simulink library "tqd"  (R2021b)
settings: Solver=VariableStepAuto  StartTime=0.0  StopTime=10.0  RelTol=1e-3
undefined symbols (not defined in the file or in its folder): ATQD_APSDecReq_X_kph, ATQD_APSDecReq_Y_mps2, ATQD_APSDecReqCMD_X_kph, ATQD_APSDecReqTs_X_pct, ATQD_APSDecTimeGain_X_Deg, ATQD_APSDecTimeGain_Y_s, ATQD_APSReqLowSpd_X_Deg, ATQD_AutoHoldReleaseBPS_X_Deg, ATQD_AWDLoadTrqnsGain_X_kg, ATQD_AWDLoadTrqnsGain_Y_pct, ATQD_BOSEnBPSPosn_X_kph, ATQD_BOSMap_X_rpm, ATQD_BOSMap_Y_pct, ATQD_CreepBaseTqD_X_kph, ATQD_CreepBaseTqD_Y_Deg, ATQD_CreepBaseTqR_X_kph, ATQD_CreepBaseTqR_Y_Deg, ATQD_CreepBPSDisPosn_X_Deg, ATQD_CreepBPSDisPosnR_X_Deg, ATQD_CreepBPSEnPosn_X_Deg, ATQD_CreepBPSEnPosnR_X_Deg, ATQD_CreepDeltaTq_X_kph, ATQD_CreepIterm_X_kph, ATQD_CreepIterm_Y_kph, ATQD_CreepItermMaxLimit_X_pct, ATQD_CreepPreloadTime_X_kph, ATQD_CreepPreloadTq_X_kph, ATQD_CreepPreloadTq_Y_s, ATQD_CreepProtTq_X_Deg, ATQD_CreepPterm_X_kph, ATQD_CreepPterm_Y_kph, ATQD_ECOTqMapD_X_rpm, ATQD_ECOTqMapD_Y_pct, ATQD_EOPDTqMapDCon_X_rpm, ATQD_EOPDTqMapDCon_Y_Deg, ATQD_EstInitVehWeight_X_c, ATQD_LHMRollGenMapD_X_rpm, ATQD_LHMRollGenMapD_Y_rpm, ATQD_LHMTqMapD_X_rpm, ATQD_LHMTqMapD_Y_pct, ATQD_NL1TqMapD_X_rpm, ATQD_NL1TqMapD_Y_pct, ATQD_NOPDTqMapDCon_X_rpm, ATQD_NOPDTqMapDCon_Y_Deg, ATQD_NRMRrEDUSpRat_X_rpm, ATQD_NRMRrEDUSpRat_Y_Nm, ATQD_OPDHoldDownRelDelay_X_Deg, ATQD_OPDHoldEnSpd_X_Deg, ATQD_OPDHoldRelDetTime_X_Deg, ATQD_OPDHoldReleaseTq_X_Deg, ATQD_OrigPedTqLowLim_X_Deg, ATQD_OrigPedTqLowLim_Y_pct, ATQD_PedalMapClimbUpLim_X_rpm, ATQD_PedalMapClimbUpLim_Y_Deg, ATQD_PreLoadTq_X_s, ATQD_RollGenMapEL1_X_rpm, ATQD_RollGenMapEL1_Y_rpm, ATQD_SL1TqMapD_X_rpm, ATQD_SL1TqMapD_Y_pct, ATQD_SlideRegenTqGain_X_Gps ... (+487)
libraries: hcu_lib x83, simulink x73, tqr x1
(part 13 of 19)

== system tqd/TQD/TorqueDemand/Signal_convert/SWC2_Subsystem/Speed Setting Mode/MSA Speed Setting ON ==
  note: MSA SPEED SETTING MODE
  VVMC_MSACrlSta_enum : Inport
  "VTQD_SWC2ScrollUpSta_enum  " : Inport  Port=2
  "VTQD_SWC2ScrollDownSta_enum  " : Inport  Port=3
  VTQD_SpdLim4SetSpd_raw32 : Inport  Port=4
  VTQD_SetSpdDeltaLongFit_kph : Inport  Port=5
  VINP_Distanceunit_flg : Inport  Port=6
  VTQD_SWC2ResUpSta_flg : Inport  Port=7
  VTQD_SWC2SetDownSta_flg : Inport  Port=8
  VINP_SmartEcoModeSW_flg : Inport  Port=9
  VINP_IVIACCAdaptiveSta_flg : Inport  Port=10
  VTQD_Set2MeterSpd_flg : Inport  Port=11
  VTQD_SetRoadSpdLim_flg : Inport  Port=12
  VINP_ADASSLIFSpdLim_enum : Inport  Port=13
  VTQD_LScrollPressShort_flg : Inport  Port=14
  VVMC_MeterIndSpeed_raw32 : Inport  Port=15
  Action Port : ActionPort  InitializeStates=reset
  " 1" : Constant  Value=KTQD_MSAActiveMetSpdLoMPH_mph
  " 80" : Constant  Value=KTQD_MSAActiveMetSpdLo_kph
  1 : Constant  Value=KTQD_SetSpdDeltaShort_kph
  160 : Constant  Value=KTQD_MSAActiveMetSpdHi_kph
  2 : Constant  Value=KTQD_MSAActiveMetSpdHiMPH_mph
  3 : Constant  Value=KTQD_SetSpdDeltaLongMPH_mph
  4 : Constant  Value=KTQD_SmartEcoLimitSpd_mph
  5 : Constant  Value=KTQD_SetSpdDeltaLong_kph
  6 : Constant  Value=KTQD_SmartEcoLimitSpd_kph
  AND : Logic  AllPortsSameDT=off  OutDataTypeStr=boolean
  AND1 : Logic  AllPortsSameDT=off  OutDataTypeStr=boolean
  Cast To Single : DataTypeConversion  OutDataTypeStr=int8
  Delta Long Fit Base : Constant  Value=KTQD_SetSpdDeltaLongFit_kph
  KTQD_ISATestSW_flg : Constant  Value=KTQD_ISATestSW_flg
  MSA : Stateflow chart  TreatAsAtomicUnit=on
      settings: PortSchema="{\"entries\":[{\"content\":{\"sides\":[{\"content\":{\"connectorIds\":[\"In9\",\"In6\",\"In3\",\"In5\",\"In7\",\"In8\",\"In1\",\"In2\",\"In12\",\"In13\",\"In14\",\"In10\",\"In11\",\"In4\"]},\"type\":\"ConnectorPlacement.EquallySpacedRectSide\",\"uuid\":\"4fee65fe-2e32-4dfc-9c8c-ef7087e97952\"},{\"content\":{\"connectorIds\":[\"Out1\"],\"side\":\"RIGHT\"},\"type\":\"ConnectorPlacement.EquallySpacedRectSide\",\"uuid\":\"8d915692-cb0b-4a06-a57e-690cea51e532\"},{\"content\":{\"connectorIds\":[],\"side\":\"TOP\"},\"type\":\"ConnectorPlacement.EquallySpacedRectSide\",\"uuid\":\"3fa43362-4ddf-4693-9d82-d4f790f00c9c\"}]},\"type\":\"ConnectorPlacement.EquallySpacedConnector\",\"uuid\":\"c1a6cfdc-58f2-45b0-af62-575976a00cf2\"}],\"packageUris\":[\"http://schema.mathworks.com/mf0/Connector/R2020b\"],\"version\":\"1.0\"}"
  MSASetSpd_241018 : Stateflow chart  TreatAsAtomicUnit=on
  ONE : Constant  Value=ONE_INT
  Relational Operator2 : RelationalOperator  Operator===  OutDataTypeStr=boolean  RndMeth=Simplest
  Relational Operator4 : RelationalOperator  Operator===  OutDataTypeStr=boolean  RndMeth=Simplest
  Round : Rounding  Operator=round
  Specific_STATE_ChangeToOFF : Stateflow chart  TreatAsAtomicUnit=on
  Switch{,1..5,7} (7 alike) : Switch  Criteria=u2 > Threshold
  standby : Constant  Value=ENUM_ADASMSASTA_STANDBY
  standby1 : Constant  Value=KTQD_MSASetSpdSource_flg
  zero : Constant  Value=ZERO_INT
  VSCP_MSASetSpd_kph : Outport
  wires:
  VTQD_SpdLim4SetSpd_raw32/1 -> [VTQD_SpdLim4SetSpd_raw32]
  Delta Long Fit Base/1 -> MSA/11(KTQD_SetSpdDeltaLongFit_kph)
  Switch2/1 -> [VTQD_MSAActiveMetSpdHi_raw32]  "VTQD_MSAActiveMetSpdHi_raw32"
  Switch3/1 -> [VTQD_MSAActiveMetSpdLo_raw32]  "VTQD_MSAActiveMetSpdLo_raw32"
  VVMC_MSACrlSta_enum/1 -> [VVMC_MSACrlSta_enum]
  1/1 -> MSA/2(KTQD_SetSpdDeltaShort_kph)
  "VTQD_SWC2ScrollDownSta_enum  "/1 -> [VTQD_SWC2ScrollDownSta_enum]
  "VTQD_SWC2ScrollUpSta_enum  "/1 -> [VTQD_SWC2ScrollUpSta_enum]
  Specific_STATE_ChangeToOFF/1(VTQD_ChangeToOFF_flg) -> [VTQD_ChangeToOFF_flg]
  [VVMC_MSACrlSta_enum] -> Specific_STATE_ChangeToOFF/1(VINP_MSACrlSta_enum)
  AND1/1 -> Switch1/2
  zero/1 -> Relational Operator4/2
  standby/1 -> Relational Operator2/2
  ONE/1 -> Switch1/1
  Cast To Single/1 -> Relational Operator4/1, Switch1/3
  Relational Operator2/1 -> AND1/1
  [VVMC_MSACrlSta_enum] -> Relational Operator2/1
  Relational Operator4/1 -> AND1/2
  Switch1/1 -> VSCP_MSASetSpd_kph/1
  [VINP_Distanceunit_flg] -> Switch2/2
  VINP_Distanceunit_flg/1 -> [VINP_Distanceunit_flg]
  [VINP_Distanceunit_flg] -> Switch3/2
  " 80"/1 -> Switch3/3
  " 1"/1 -> Switch3/1
  [VINP_Distanceunit_flg] -> Switch4/2
  5/1 -> Switch4/3
  3/1 -> Switch4/1
  Round/1 -> Cast To Single/1
  VINP_SmartEcoModeSW_flg/1 -> [VINP_SmartEcoModeSW_flg]
  [VINP_SmartEcoModeSW_flg] -> Switch/2
  160/1 -> Switch/3
  Switch/1 -> Switch2/3
  [VINP_SmartEcoModeSW_flg] -> Switch5/2
  2/1 -> Switch5/3
  Switch5/1 -> Switch2/1
  4/1 -> Switch5/1
  6/1 -> Switch/1
  [VTQD_ChangeToOFF_flg] -> MSA/3(VTQD_ChangeToOFF_flg)
  [VVMC_MSACrlSta_enum] -> MSASetSpd_241018/1(VVMC_MSACrlSta_enum)
  AND/1 -> MSASetSpd_241018/2(VINP_IVIACCAdaptiveSta_flg)
  KTQD_ISATestSW_flg/1 -> AND/2
  [VTQD_SpdLim4SetSpd_raw32] -> MSASetSpd_241018/3(VTQD_SpdLim4SetSpd_raw32)
  [VTQD_MSAActiveMetSpdHi_raw32] -> MSASetSpd_241018/4(VTQD_MSAActiveMetSpdHi_raw32)
  [VTQD_MSAActiveMetSpdLo_raw32] -> MSASetSpd_241018/5(VTQD_MSAActiveMetSpdLo_raw32)
  [VTQD_SWC2ScrollUpSta_enum] -> MSASetSpd_241018/7(VTQD_SWC2ScrollUpSta_enum)
  [VTQD_SWC2ScrollDownSta_enum] -> MSASetSpd_241018/8(VTQD_SWC2ScrollDownSta_enum)
  [VINP_Distanceunit_flg] -> MSASetSpd_241018/11(VINP_Distanceunit_flg)
  MSASetSpd_241018/1(VTQD_MSASetSpd_raw32) -> [VTQD_MSASetSpd_raw32]  "VTQD_MSASetSpd_raw32"
  standby1/1 -> Switch7/2
  [VTQD_MSASetSpd_raw32] -> Switch7/1
  Switch7/1 -> Round/1
  VTQD_SetSpdDeltaLongFit_kph/1 -> [VTQD_SetSpdDeltaLongFit_kph]
  VTQD_SWC2ResUpSta_flg/1 -> [VTQD_SWC2ResUpSta_flg]
  Switch4/1 -> [VTQD_SetSpdDeltaLong_kph]  "VTQD_SetSpdDeltaLong_kph"
  VTQD_SWC2SetDownSta_flg/1 -> [VTQD_SWC2SetDownSta_flg]
  VINP_IVIACCAdaptiveSta_flg/1 -> [VINP_IVIACCAdaptiveSta_flg]
  [VINP_IVIACCAdaptiveSta_flg] -> AND/1
  VTQD_Set2MeterSpd_flg/1 -> [VTQD_Set2MeterSpd_flg]
  [VTQD_Set2MeterSpd_flg] -> MSASetSpd_241018/6(VTQD_Set2MeterSpd_flg)
  VTQD_SetRoadSpdLim_flg/1 -> [VTQD_SetRoadSpdLim_flg]
  [VTQD_SetRoadSpdLim_flg] -> MSASetSpd_241018/10(VTQD_SetRoadSpdLim_flg)
  VINP_ADASSLIFSpdLim_enum/1 -> [VINP_ADASSLIFSpdLim_enum]
  [VINP_ADASSLIFSpdLim_enum] -> MSASetSpd_241018/12(VTQD_ADASSLIFSpdLimDet_flg)
  VTQD_LScrollPressShort_flg/1 -> [VTQD_LScrollPressShort_flg]
  [VTQD_LScrollPressShort_flg] -> MSASetSpd_241018/13(VTQD_LScrollPressShort_flg)
  VVMC_MeterIndSpeed_raw32/1 -> [VVMC_MeterIndSpeed_raw32]
  [VVMC_MeterIndSpeed_raw32] -> MSASetSpd_241018/14(VVMC_MeterIndSpeed_raw32)
  [VTQD_SetSpdDeltaLong_kph] -> MSASetSpd_241018/9(VTQD_SetSpdDeltaLong_raw32)
  [VVMC_MSACrlSta_enum] -> MSA/9(VVMC_MSACrlSta_enum)
  [VTQD_SpdLim4SetSpd_raw32] -> MSA/6(VVMC_MeterIndSpeed_raw32)
  [VINP_Distanceunit_flg] -> MSA/5(VINP_Distanceunit_flg)
  [VTQD_MSAActiveMetSpdHi_raw32] -> MSA/7(KTQD_MSAActiveMetSpdHi_raw32)
  [VTQD_MSAActiveMetSpdLo_raw32] -> MSA/8(KTQD_MSAActiveMetSpdLo_raw32)
  [VTQD_SetSpdDeltaLong_kph] -> MSA/1(KTQD_SetSpdDeltaLong_kph)
  [VTQD_SWC2ScrollUpSta_enum] -> MSA/12(VTQD_SWC2ScrollUpSta_enum)
  [VTQD_SWC2ResUpSta_flg] -> MSA/13(VTQD_SWC2ResUpSta_flg)
  [VTQD_SWC2SetDownSta_flg] -> MSA/14(VTQD_SWC2SetDownSta_flg)
  [VTQD_SetSpdDeltaLongFit_kph] -> MSA/10(VTQD_SetSpdDeltaLongFit_kph)
  [VTQD_SWC2ScrollDownSta_enum] -> MSA/4(VTQD_SWC2ScrollDownSta_enum)
  MSA/1(VTQD_MSASetSpd_kph) -> [VTQD_MSASetSpd_kph]  "VTQD_MSASetSpd_kph"
  [VTQD_MSASetSpd_kph] -> Switch7/3

== system tqd/TQD/TorqueDemand/Signal_convert/SWC2_Subsystem/Speed Setting Mode/SWC2ScrollDownSta ==
  note: Long press or Short press
  INPUT : Inport
  task_time_s : Inport  Port=2
  AND : Logic  AllPortsSameDT=off  OutDataTypeStr=boolean
  AND1 : Logic  AllPortsSameDT=off  OutDataTypeStr=boolean
  Constant1 : Constant  Value=ENUM_SWCBOTTONPRESS_LONGPRESS
  Constant2 : Constant  Value=KTQD_ScrollDownShortPLim_s
  Constant3 : Constant  Value=KTQD_ScrollDownLongPLim_s
  Constant7 : Constant  Value=ENUM_SWCBOTTONPRESS_SHORTPRESS
  Constant8 : Constant  Value=ENUM_SWCBOTTONPRESS_NOPRESS
  Delay : Delay  DelayLength=1
  DelayEnable_LONG_PRESS1 : hcu_lib/Basic_Blocks/DelayEnable
  DelayEnable_SHORT_PRESS1 : hcu_lib/Basic_Blocks/DelayEnable
  Detect Decrease : simulink/Logic and Bit Operations/Detect Decrease  vinit=0.0  OutDataTypeStr=boolean
  Detect Decrease4 : simulink/Logic and Bit Operations/Detect Decrease  vinit=0.0  OutDataTypeStr=boolean
  NOT : Logic  Operator=NOT  AllPortsSameDT=off  OutDataTypeStr=boolean
  NOT1 : Logic  Operator=NOT  AllPortsSameDT=off  OutDataTypeStr=boolean
  SR_Latch : hcu_lib/Basic_Blocks/SR_Latch
  Switch : Switch  Criteria=u2 ~= 0
  Switch3 : Switch  Criteria=u2 ~= 0
  OUTPUT : Outport
  wires:
  [Short_press_falling_Edge] -> Switch3/2
  Detect Decrease/1 -> SR_Latch/2
  [INPUT] -> Detect Decrease/1
  NOT1/1 -> AND1/2
  SR_Latch/1 -> NOT1/1
  [INPUT] -> AND1/1
  AND1/1 -> DelayEnable_SHORT_PRESS1/1
  [Long_press_falling_edge] -> SR_Latch/1
  [INPUT] -> AND/1
  AND/1 -> DelayEnable_LONG_PRESS1/1
  NOT/1 -> AND/2
  Delay/1 -> NOT/1
  [Long_press_falling_edge] -> Delay/1
  INPUT/1 -> [INPUT]
  task_time_s/1 -> [task_time_s]
  DelayEnable_LONG_PRESS1/1 -> [Long_press_falling_edge]
  Switch3/1 -> Switch/3
  DelayEnable_SHORT_PRESS1/1 -> Detect Decrease4/1
  Constant3/1 -> DelayEnable_LONG_PRESS1/2
  Constant2/1 -> DelayEnable_SHORT_PRESS1/2
  [task_time_s] -> DelayEnable_SHORT_PRESS1/3
  [task_time_s] -> DelayEnable_LONG_PRESS1/3
  Detect Decrease4/1 -> [Short_press_falling_Edge]
  [Long_press_falling_edge] -> Switch/2
  Constant7/1 -> Switch3/1
  Constant1/1 -> Switch/1
  Constant8/1 -> Switch3/3
  Switch/1 -> OUTPUT/1

== system tqd/TQD/TorqueDemand/Signal_convert/SWC2_Subsystem/Speed Setting Mode/SWC2ScrollUpSta ==
  note: Long press or Short press
  INPUT : Inport
  task_time_s : Inport  Port=2
  AND : Logic  AllPortsSameDT=off  OutDataTypeStr=boolean
  AND1 : Logic  AllPortsSameDT=off  OutDataTypeStr=boolean
  Constant2 : Constant  Value=KTQD_ScrollUpShortPLim_s
  Constant3 : Constant  Value=KTQD_ScrollUpLongPLim_s
  Constant4 : Constant  Value=ENUM_SWCBOTTONPRESS_LONGPRESS
  Constant5 : Constant  Value=ENUM_SWCBOTTONPRESS_SHORTPRESS
  Constant6 : Constant  Value=ENUM_SWCBOTTONPRESS_NOPRESS
  Delay : Delay  DelayLength=1
  DelayEnable_LONG_PRESS1 : hcu_lib/Basic_Blocks/DelayEnable
  DelayEnable_SHORT_PRESS1 : hcu_lib/Basic_Blocks/DelayEnable
  Detect Decrease : simulink/Logic and Bit Operations/Detect Decrease  vinit=0.0  OutDataTypeStr=boolean
  Detect Decrease4 : simulink/Logic and Bit Operations/Detect Decrease  vinit=0.0  OutDataTypeStr=boolean
  NOT : Logic  Operator=NOT  AllPortsSameDT=off  OutDataTypeStr=boolean
  NOT1 : Logic  Operator=NOT  AllPortsSameDT=off  OutDataTypeStr=boolean
  SR_Latch : hcu_lib/Basic_Blocks/SR_Latch
  Switch : Switch  Criteria=u2 ~= 0
  Switch3 : Switch  Criteria=u2 ~= 0
  OUTPUT : Outport
  wires:
  [Short_press_falling_Edge] -> Switch3/2
  Detect Decrease/1 -> SR_Latch/2
  [INPUT] -> Detect Decrease/1
  NOT1/1 -> AND1/2
  SR_Latch/1 -> NOT1/1
  [INPUT] -> AND1/1
  AND1/1 -> DelayEnable_SHORT_PRESS1/1
  [Long_press_falling_edge] -> SR_Latch/1
  [INPUT] -> AND/1
  AND/1 -> DelayEnable_LONG_PRESS1/1
  NOT/1 -> AND/2
  Delay/1 -> NOT/1
  [Long_press_falling_edge] -> Delay/1
  INPUT/1 -> [INPUT]
  task_time_s/1 -> [task_time_s]
  DelayEnable_LONG_PRESS1/1 -> [Long_press_falling_edge]
  Switch3/1 -> Switch/3
  DelayEnable_SHORT_PRESS1/1 -> Detect Decrease4/1
  Constant3/1 -> DelayEnable_LONG_PRESS1/2
  Constant2/1 -> DelayEnable_SHORT_PRESS1/2
  [task_time_s] -> DelayEnable_SHORT_PRESS1/3
  [task_time_s] -> DelayEnable_LONG_PRESS1/3
  Detect Decrease4/1 -> [Short_press_falling_Edge]
  [Long_press_falling_edge] -> Switch/2
  Constant5/1 -> Switch3/1
  Constant4/1 -> Switch/1
  Constant6/1 -> Switch3/3
  Switch/1 -> OUTPUT/1

== system tqd/TQD/TorqueDemand/Signal_convert/SWC_Subsystem/Speed Setting Mode/ACC Speed Setting ON ==
  note: ACC SPEED SETTING MODE
  VTQD_SWCResUpSta_flg : Inport
  VTQD_SWCSetDownSta_flg : Inport  Port=2
  task_time_s : Inport  Port=3
  VVMC_LVDAACCStatusInformation_flg : Inport  Port=4
  VVMC_ACCObjDist_m : Inport  Port=5
  VVMC_MeterIndSpeed_raw32 : Inport  Port=6
  VINP_ADASACCSta_enum : Inport  Port=7
  VINP_Distanceunit_flg : Inport  Port=8
  VINP_SmartEcoModeSW_flg : Inport  Port=9
  VVMC_SetACCDisableAPS_flg : Inport  Port=10
  Action Port : ActionPort  InitializeStates=reset  ActionPortLabel=if(u1 ~= 0)
  " 20" : Constant  Value=KTQD_ACCActiveMetSpdLoMPH_mph
  " 30kph" : Constant  Value=KTQD_ACCActiveMetSpdLo_kph
  0 : Constant  Value=KTQD_AllowSetSpdOvrd_flg
  1 : Constant  Value=KTQD_AllowSetSpdOvrdVal_flg
  1.1s : Constant  Value=KTQD_SetSpdLongPLim_s
  105 : Constant  Value=KTQD_ACCActiveMetSpdHiMPH_mph
  10kph1 : Constant  Value=KTQD_AllowSetSpdSpd_kph
  180kph : Constant  Value=KTQD_ACCActiveMetSpdHi_kph
  2 : Constant  Value=KTQD_SmartEcoLimitSpd_kph
  20m : Constant  Value=KVMC_AllowSetSpdDist_m
  2m : Constant  Value=KVMC_NotAllowSetSpdDist_m
  3 : Constant  Value=KTQD_SmartEcoLimitSpd_kph
  5 : Constant  Value=KTQD_SetSpdDeltaLongMPH_mph
  5kph : Constant  Value=KTQD_SetSpdDeltaLong_kph
  ACCSetSpd_Chart_W : Stateflow chart  TreatAsAtomicUnit=on
      settings: PortSchema="{\"entries\":[{\"content\":{\"sides\":[{\"content\":{\"connectorIds\":[\"In1\",\"In2\",\"In3\",\"In4\",\"In5\",\"In6\",\"In7\",\"In8\",\"In12\",\"In9\",\"In10\",\"In11\"]},\"type\":\"ConnectorPlacement.EquallySpacedRectSide\",\"uuid\":\"61ce72b2-2f56-4065-9e06-1345412a8c86\"},{\"content\":{\"connectorIds\":[\"Out1\"],\"side\":\"RIGHT\"},\"type\":\"ConnectorPlacement.EquallySpacedRectSide\",\"uuid\":\"4594d6d3-f7cd-4711-8df0-9a0a2c5601b5\"},{\"content\":{\"connectorIds\":[],\"side\":\"TOP\"},\"type\":\"ConnectorPlacement.EquallySpacedRectSide\",\"uuid\":\"a8857ab2-f9b0-4737-b2f3-522f42c1ada3\"}]},\"type\":\"ConnectorPlacement.EquallySpacedConnector\",\"uuid\":\"0a7f8e6a-9c19-454d-bd26-d3d8923cc49e\"}],\"packageUris\":[\"http://schema.mathworks.com/mf0/Connector/R2020b\"],\"version\":\"1.0\"}"
  AND : Logic  AllPortsSameDT=off  OutDataTypeStr=boolean
  AND1 : Logic  AllPortsSameDT=off  OutDataTypeStr=boolean
  Cast To Single : DataTypeConversion  OutDataTypeStr=int8
  Data Type Conversion : DataTypeConversion  OutDataTypeStr=uint8
  Data Type Conversion1 : DataTypeConversion  OutDataTypeStr=uint8
  Logical Operator : Logic  AllPortsSameDT=off  OutDataTypeStr=boolean
  ONE : Constant  Value=ONE_INT
  OR : Logic  Operator=OR  AllPortsSameDT=off  OutDataTypeStr=boolean
  Product : Product
  Relational Operator : RelationalOperator  Operator=<=  OutDataTypeStr=boolean  RndMeth=Simplest
  Relational Operator1 : RelationalOperator  Operator=>  OutDataTypeStr=boolean  RndMeth=Simplest
  Relational Operator2 : RelationalOperator  Operator===  OutDataTypeStr=boolean  RndMeth=Simplest
  Relational Operator3 : RelationalOperator  OutDataTypeStr=boolean  RndMeth=Simplest
  Relational Operator4 : RelationalOperator  Operator===  OutDataTypeStr=boolean  RndMeth=Simplest
  Round : Rounding  Operator=round
  Switch{,1..6} (7 alike) : Switch  Criteria=u2 > Threshold
  standby : Constant  Value=ENUM_ADASACCSTA_STANDBY
  zero : Constant  Value=ZERO_INT
  zero1 : Constant  Value=KPH2MPH
  VTQD_ACCSetSpd_kph : Outport
  VTQD_SWCAllowSetSpd_flg : Outport  Port=2
  wires:
  VVMC_LVDAACCStatusInformation_flg/1 -> ACCSetSpd_Chart_W/10(VVMC_LVDAACCStatusInformation_flg)
  1.1s/1 -> ACCSetSpd_Chart_W/9(KTQD_SetSpdLongPLim_s)
  task_time_s/1 -> ACCSetSpd_Chart_W/12(task_time_s)
  Switch4/1 -> ACCSetSpd_Chart_W/8(KTQD_SetSpdDeltaLong_kph)
  Switch3/1 -> ACCSetSpd_Chart_W/7(KTQD_ACCActiveMetSpdLo_raw32)
  VVMC_MeterIndSpeed_raw32/1 -> ACCSetSpd_Chart_W/4(VVMC_MeterIndSpeed_raw32), [VVMC_MeterIndSpeed_raw32]
  VTQD_SWCSetDownSta_flg/1 -> ACCSetSpd_Chart_W/3(VTQD_SWCSetDownSta_flg)
  VTQD_SWCResUpSta_flg/1 -> ACCSetSpd_Chart_W/2(VTQD_SWCResUpSta_flg)
  VINP_ADASACCSta_enum/1 -> [VINP_ADASACCSta_enum], ACCSetSpd_Chart_W/1(VINP_ADASACCSta_enum)
  VVMC_ACCObjDist_m/1 -> Relational Operator/1, Relational Operator1/1
  20m/1 -> Relational Operator/2
  2m/1 -> Relational Operator1/2
  Relational Operator/1 -> AND/1
  Relational Operator1/1 -> AND/2
  [VVMC_MeterIndSpeed_raw32] -> Relational Operator3/1
  10kph1/1 -> Relational Operator3/2
  AND/1 -> OR/1
  Relational Operator3/1 -> OR/2
  Switch/1 -> VTQD_SWCAllowSetSpd_flg/1, [VTQD_AllowSetSpd_flg]  "VTQD_SWCAllowSetSpd_flg"
  0/1 -> Switch/2
  1/1 -> Switch/1
  [VTQD_AllowSetSpd_flg] -> ACCSetSpd_Chart_W/11(VTQD_AllowSetSpd_flg)
  Cast To Single/1 -> Relational Operator4/1, Switch1/3
  Switch1/1 -> VTQD_ACCSetSpd_kph/1
  [VINP_ADASACCSta_enum] -> Relational Operator2/1
  AND1/1 -> Switch1/2
  ONE/1 -> Switch1/1
  standby/1 -> Relational Operator2/2
  zero/1 -> Relational Operator4/2
  Relational Operator2/1 -> AND1/1
  Relational Operator4/1 -> AND1/2
  VINP_Distanceunit_flg/1 -> [VINP_Distanceunit_flg]
  [VINP_Distanceunit_flg] -> Switch3/2
  " 30kph"/1 -> Switch3/3
  " 20"/1 -> Switch3/1
  [VINP_Distanceunit_flg] -> Switch4/2
  5kph/1 -> Switch4/3
  5/1 -> Switch4/1
  [VINP_Distanceunit_flg] -> ACCSetSpd_Chart_W/6(VINP_Distanceunit_flg)
  Round/1 -> Cast To Single/1
  ACCSetSpd_Chart_W/1(VTQD_ACCSetSpd_kph) -> Round/1
  VINP_SmartEcoModeSW_flg/1 -> [VINP_SmartEcoModeSW_flg]
  180kph/1 -> Switch5/3
  2/1 -> Product/1
  zero1/1 -> Product/2
  Product/1 -> Data Type Conversion/1
  105/1 -> Switch6/3
  Switch5/1 -> Switch2/3
  Switch6/1 -> Switch2/1
  3/1 -> Data Type Conversion1/1
  [VINP_Distanceunit_flg] -> Switch2/2
  [VINP_SmartEcoModeSW_flg] -> Switch6/2
  [VINP_SmartEcoModeSW_flg] -> Switch5/2
  Data Type Conversion/1 -> Switch6/1
  Switch2/1 -> ACCSetSpd_Chart_W/5(KTQD_ACCActiveMetSpdHi_raw32)
  Data Type Conversion1/1 -> Switch5/1
  OR/1 -> Logical Operator/1
  Logical Operator/1 -> Switch/3
  VVMC_SetACCDisableAPS_flg/1 -> Logical Operator/2

== system tqd/TQD/TorqueDemand/Signal_convert/SWC_Subsystem/Speed Setting Mode/CC Speed Setting ON ==
  note: CC SPEED SETTING MODE
  VVMC_CCCtrlSta_enum : Inport
  "VTQD_SWCResUpPress_enum  " : Inport  Port=2
  "VTQD_SWCSetDownPress_enum  " : Inport  Port=3
  VVMC_MeterIndSpeed_raw32 : Inport  Port=4
  VTQD_SetSpdDeltaLongFit_kph : Inport  Port=5
  VINP_Distanceunit_flg : Inport  Port=6
  VINP_SmartEcoModeSW_flg : Inport  Port=7
  Action Port : ActionPort  InitializeStates=reset
  " 1" : Constant  Value=KTQD_CCActiveMetSpdLo_kph
  " 2" : Constant  Value=KTQD_CCActiveMetSpdLoMPH_mph
  1 : Constant  Value=KTQD_SetSpdDeltaLongFit_kph
  2 : Constant  Value=KTQD_SetSpdDeltaShort_kph
  3 : Constant  Value=KTQD_SmartEcoLimitSpd_kph
  4 : Constant  Value=KTQD_SetSpdDeltaLong_kph
  5 : Constant  Value=KTQD_SmartEcoLimitSpd_kph
  6 : Constant  Value=KTQD_SetSpdDeltaLongMPH_mph
  7 : Constant  Value=KTQD_CCActiveMetSpdHi_kph
  8 : Constant  Value=KTQD_CCActiveMetSpdHiMPH_mph
  AND1 : Logic  AllPortsSameDT=off  OutDataTypeStr=boolean
  CC Speed Setting Mode : Stateflow chart  TreatAsAtomicUnit=on
      settings: PortSchema="{\"entries\":[{\"content\":{\"sides\":[{\"content\":{\"connectorIds\":[\"In5\",\"In12\",\"In4\",\"In3\",\"In9\",\"In6\",\"In7\",\"In8\",\"In1\",\"In2\",\"In11\",\"In10\"]},\"type\":\"ConnectorPlacement.EquallySpacedRectSide\",\"uuid\":\"331c8dfa-4564-419d-9323-fdbf8561d50b\"},{\"content\":{\"connectorIds\":[\"Out1\",\"Out2\"],\"side\":\"RIGHT\"},\"type\":\"ConnectorPlacement.EquallySpacedRectSide\",\"uuid\":\"71cb1444-7708-4b6f-91dd-d8a1c8c14ea8\"},{\"content\":{\"connectorIds\":[],\"side\":\"TOP\"},\"type\":\"ConnectorPlacement.EquallySpacedRectSide\",\"uuid\":\"6ecf38bb-d171-491a-a8b2-073f135e7039\"}]},\"type\":\"ConnectorPlacement.EquallySpacedConnector\",\"uuid\":\"fc3afa97-6e6e-4933-9aff-7c8f8cbb1702\"}],\"packageUris\":[\"http://schema.mathworks.com/mf0/Connector/R2020b\"],\"version\":\"1.0\"}"
  Cast To Single : DataTypeConversion  OutDataTypeStr=int8
  Data Type Conversion : DataTypeConversion  OutDataTypeStr=uint8
  Data Type Conversion1 : DataTypeConversion  OutDataTypeStr=uint8
  ONE : Constant  Value=ONE_INT
  Product : Product
  Relational Operator2 : RelationalOperator  Operator===  OutDataTypeStr=boolean  RndMeth=Simplest
  Relational Operator4 : RelationalOperator  Operator===  OutDataTypeStr=boolean  RndMeth=Simplest
  Round : Rounding  Operator=round
  Specific_STATE_ChangeToSTANDBY : Stateflow chart  TreatAsAtomicUnit=on
  Switch{1..6} (6 alike) : Switch  Criteria=u2 > Threshold
  standby : Constant  Value=ENUM_ADASCCSTA_STANDBY
  zero : Constant  Value=ZERO_INT
  zero1 : Constant  Value=KPH2MPH
  VTQD_CCSetSpd_kph : Outport
  VTQD_SWCCCSpdResetFinish_flg : Outport  Port=2
  wires:
  "VTQD_SWCSetDownPress_enum  "/1 -> CC Speed Setting Mode/10(VTQD_SWCSetDownPress_enum)
  [VTQD_ChangeToSTANDBY_flg] -> CC Speed Setting Mode/12(VTQD_ChangeToSTANDBY_flg)
  Specific_STATE_ChangeToSTANDBY/1(VTQD_CCChangeToSTANDBY_flg) -> [VTQD_ChangeToSTANDBY_flg]  "VTQD_CCChangeToSTANDBY_flg"
  [VVMC_CCCtrlSta_enum] -> Specific_STATE_ChangeToSTANDBY/1(VVMC_CCCtrlSta_enum)
  "VTQD_SWCResUpPress_enum  "/1 -> CC Speed Setting Mode/11(VTQD_SWCResUpPress_enum)
  VVMC_CCCtrlSta_enum/1 -> CC Speed Setting Mode/5(VVMC_CCCtrlSta_enum), [VVMC_CCCtrlSta_enum]
  2/1 -> CC Speed Setting Mode/2(KTQD_SetSpdDeltaShort_kph)
  Switch3/1 -> CC Speed Setting Mode/8(KTQD_CCActiveMetSpdLo_raw32)
  Switch4/1 -> CC Speed Setting Mode/1(KTQD_SetSpdDeltaLong_kph)
  CC Speed Setting Mode/2(VTQD_CCSpdResetFinish_flg) -> VTQD_SWCCCSpdResetFinish_flg/1  "VTQD_SWCCCSpdResetFinish_flg"
  VTQD_SetSpdDeltaLongFit_kph/1 -> CC Speed Setting Mode/4(VTQD_SetSpdDeltaLongFit_kph)
  1/1 -> CC Speed Setting Mode/3(KTQD_SetSpdDeltaLongFit_kph)
  VVMC_MeterIndSpeed_raw32/1 -> CC Speed Setting Mode/9(VVMC_MeterIndSpeed_raw32)
  Cast To Single/1 -> Relational Operator4/1, Switch1/3
  Switch1/1 -> VTQD_CCSetSpd_kph/1
  [VVMC_CCCtrlSta_enum] -> Relational Operator2/1
  AND1/1 -> Switch1/2
  ONE/1 -> Switch1/1
  standby/1 -> Relational Operator2/2
  zero/1 -> Relational Operator4/2
  Relational Operator2/1 -> AND1/1
  Relational Operator4/1 -> AND1/2
  VINP_Distanceunit_flg/1 -> [VINP_Distanceunit_flg]
  [VINP_Distanceunit_flg] -> Switch3/2
  " 1"/1 -> Switch3/3
  " 2"/1 -> Switch3/1
  [VINP_Distanceunit_flg] -> Switch4/2
  4/1 -> Switch4/3
  6/1 -> Switch4/1
  [VINP_Distanceunit_flg] -> CC Speed Setting Mode/6(VINP_Distanceunit_flg)
  Round/1 -> Cast To Single/1
  CC Speed Setting Mode/1(VTQD_CCSetSpd_kph) -> Round/1
  Switch5/1 -> Switch2/3
  [VINP_Distanceunit_flg] -> Switch2/2
  [VINP_SmartEcoModeSW_flg] -> Switch5/2
  3/1 -> Data Type Conversion1/1
  [VINP_SmartEcoModeSW_flg] -> Switch6/2
  Switch6/1 -> Switch2/1
  Product/1 -> Data Type Conversion/1
  Data Type Conversion/1 -> Switch6/1
  zero1/1 -> Product/2
  5/1 -> Product/1
  Switch2/1 -> CC Speed Setting Mode/7(KTQD_CCActiveMetSpdHi_raw32)
  VINP_SmartEcoModeSW_flg/1 -> [VINP_SmartEcoModeSW_flg]
  7/1 -> Switch5/3
  8/1 -> Switch6/3
  Data Type Conversion1/1 -> Switch5/1

== system tqd/TQD/TorqueDemand/Signal_convert/SWC_Subsystem/Speed Setting Mode/Else Speed Setting On ==
  In : Inport
  Action Port : ActionPort  ActionPortLabel=else
  Data Type Conversion : DataTypeConversion
  Out : Outport
  wires:
  Data Type Conversion/1 -> Out/1
  In/1 -> Data Type Conversion/1

== system tqd/TQD/TorqueDemand/Signal_convert/SWC_Subsystem/Speed Setting Mode/ISA Speed Setting ON ==
  VINP_ADASVehSpdLim_kph : Inport
  VINP_SmartEcoModeSW_flg : Inport  Port=2
  Action Port : ActionPort
  8 : Constant  Value=KTQD_SmartEcoLimitSpd_kph
  Data Type Conversion : DataTypeConversion
  Min : MinMax  Inputs=2
  Switch : Switch  Criteria=u2 > Threshold
  VTQD_ISASetSpd_kph : Outport
  wires:
  Min/1 -> Switch/1
  Switch/1 -> Data Type Conversion/1
  VINP_ADASVehSpdLim_kph/1 -> Min/2, Switch/3
  VINP_SmartEcoModeSW_flg/1 -> Switch/2
  8/1 -> Min/1
  Data Type Conversion/1 -> VTQD_ISASetSpd_kph/1

== system tqd/TQD/TorqueDemand/Signal_convert/SWC_Subsystem/Speed Setting Mode/MSA Speed Setting ON ==
  note: MSA SPEED SETTING MODE
  VVMC_MSACrlSta_enum : Inport
  "VTQD_SWCResUpPress_enum  " : Inport  Port=2
  "VTQD_SWCSetDownPress_enum  " : Inport  Port=3
  VVMC_MeterIndSpeed_raw32 : Inport  Port=4
  VTQD_SetSpdDeltaLongFit_kph : Inport  Port=5
  VINP_Distanceunit_flg : Inport  Port=6
  VINP_SmartEcoModeSW_flg : Inport  Port=7
  Action Port : ActionPort  InitializeStates=reset  ActionPortLabel=elseif( u3~= 0)
  " 1" : Constant  Value=KTQD_MSAActiveMetSpdLoMPH_mph
  " 80" : Constant  Value=KTQD_MSAActiveMetSpdLo_kph
  1 : Constant  Value=KTQD_SetSpdDeltaShort_kph
  160 : Constant  Value=KTQD_MSAActiveMetSpdHi_kph
  2 : Constant  Value=KTQD_SmartEcoLimitSpd_kph
  3 : Constant  Value=KTQD_SetSpdDeltaLongMPH_mph
  4 : Constant  Value=KTQD_SmartEcoLimitSpd_kph
  5 : Constant  Value=KTQD_SetSpdDeltaLong_kph
  6 : Constant  Value=KTQD_MSAActiveMetSpdHiMPH_mph
  AND1 : Logic  AllPortsSameDT=off  OutDataTypeStr=boolean
  Cast To Single : DataTypeConversion  OutDataTypeStr=int8
  Data Type Conversion : DataTypeConversion  OutDataTypeStr=uint8
  Data Type Conversion1 : DataTypeConversion  OutDataTypeStr=uint8
  Delta Long Fit Base : Constant  Value=KTQD_SetSpdDeltaLongFit_kph
  MSA : Stateflow chart  TreatAsAtomicUnit=on
      settings: PortSchema="{\"entries\":[{\"content\":{\"sides\":[{\"content\":{\"connectorIds\":[\"In9\",\"In6\",\"In5\",\"In4\",\"In7\",\"In8\",\"In1\",\"In2\",\"In12\",\"In10\",\"In11\",\"In3\"]},\"type\":\"ConnectorPlacement.EquallySpacedRectSide\",\"uuid\":\"4fee65fe-2e32-4dfc-9c8c-ef7087e97952\"},{\"content\":{\"connectorIds\":[\"Out1\"],\"side\":\"RIGHT\"},\"type\":\"ConnectorPlacement.EquallySpacedRectSide\",\"uuid\":\"8d915692-cb0b-4a06-a57e-690cea51e532\"},{\"content\":{\"connectorIds\":[],\"side\":\"TOP\"},\"type\":\"ConnectorPlacement.EquallySpacedRectSide\",\"uuid\":\"3fa43362-4ddf-4693-9d82-d4f790f00c9c\"}]},\"type\":\"ConnectorPlacement.EquallySpacedConnector\",\"uuid\":\"c1a6cfdc-58f2-45b0-af62-575976a00cf2\"}],\"packageUris\":[\"http://schema.mathworks.com/mf0/Connector/R2020b\"],\"version\":\"1.0\"}"
  ONE : Constant  Value=ONE_INT
  Product : Product
  Relational Operator2 : RelationalOperator  Operator===  OutDataTypeStr=boolean  RndMeth=Simplest
  Relational Operator4 : RelationalOperator  Operator===  OutDataTypeStr=boolean  RndMeth=Simplest
  Round : Rounding  Operator=round
  Specific_STATE_ChangeToOFF : Stateflow chart  TreatAsAtomicUnit=on
  Switch{1..6} (6 alike) : Switch  Criteria=u2 > Threshold
  standby : Constant  Value=ENUM_ADASMSASTA_STANDBY
  zero : Constant  Value=ZERO_INT
  zero1 : Constant  Value=KPH2MPH
  VSCP_MSASetSpd_kph : Outport
  wires:
  VVMC_MeterIndSpeed_raw32/1 -> MSA/6(VVMC_MeterIndSpeed_raw32)
  Delta Long Fit Base/1 -> MSA/11(KTQD_SetSpdDeltaLongFit_kph)
  VTQD_SetSpdDeltaLongFit_kph/1 -> MSA/10(VTQD_SetSpdDeltaLongFit_kph)
  Switch3/1 -> MSA/8(KTQD_MSAActiveMetSpdLo_raw32)
  VVMC_MSACrlSta_enum/1 -> [VINP_MSACrlSta_enum], MSA/9(VVMC_MSACrlSta_enum)
  1/1 -> MSA/2(KTQD_SetSpdDeltaShort_kph)
  Switch4/1 -> MSA/1(KTQD_SetSpdDeltaLong_kph)
  [VTQD_ChangeToOFF_flg] -> MSA/5(VTQD_ChangeToOFF_flg)
  "VTQD_SWCSetDownPress_enum  "/1 -> MSA/3(VTQD_SWCSetDownPress_enum)
  "VTQD_SWCResUpPress_enum  "/1 -> MSA/12(VTQD_SWCResUpPress_enum)
  Specific_STATE_ChangeToOFF/1(VTQD_ChangeToOFF_flg) -> [VTQD_ChangeToOFF_flg]  "VTQD_ChangeToOFF_flg"
  [VINP_MSACrlSta_enum] -> Specific_STATE_ChangeToOFF/1(VINP_MSACrlSta_enum)
  AND1/1 -> Switch1/2
  zero/1 -> Relational Operator4/2
  standby/1 -> Relational Operator2/2
  ONE/1 -> Switch1/1
  Cast To Single/1 -> Relational Operator4/1, Switch1/3
  Relational Operator2/1 -> AND1/1
  [VINP_MSACrlSta_enum] -> Relational Operator2/1
  Relational Operator4/1 -> AND1/2
  Switch1/1 -> VSCP_MSASetSpd_kph/1
  VINP_Distanceunit_flg/1 -> [VINP_Distanceunit_flg]
  [VINP_Distanceunit_flg] -> Switch3/2
  " 80"/1 -> Switch3/3
  " 1"/1 -> Switch3/1
  [VINP_Distanceunit_flg] -> Switch4/2
  5/1 -> Switch4/3
  3/1 -> Switch4/1
  [VINP_Distanceunit_flg] -> MSA/4(VINP_Distanceunit_flg)
  Round/1 -> Cast To Single/1
  MSA/1(VTQD_MSASetSpd_kph) -> Round/1
  VINP_SmartEcoModeSW_flg/1 -> [VINP_SmartEcoModeSW_flg]
  Switch2/1 -> MSA/7(KTQD_MSAActiveMetSpdHi_raw32)
  4/1 -> Product/1
  zero1/1 -> Product/2
  Switch5/1 -> Switch2/3
  Switch6/1 -> Switch2/1
  Product/1 -> Data Type Conversion/1
  2/1 -> Data Type Conversion1/1
  [VINP_Distanceunit_flg] -> Switch2/2
  [VINP_SmartEcoModeSW_flg] -> Switch6/2
  [VINP_SmartEcoModeSW_flg] -> Switch5/2
  Data Type Conversion/1 -> Switch6/1
  160/1 -> Switch5/3
  6/1 -> Switch6/3
  Data Type Conversion1/1 -> Switch5/1

== system tqd/TQD/TorqueDemand/Signal_convert/SWC_Subsystem/Speed Setting Mode/VTQD_SWCCancelP_flg ==
  INPUT : Inport
  Detect Decrease : simulink/Logic and Bit Operations/Detect Decrease  vinit=0.0  OutDataTypeStr=boolean
  Falling_edge : Outport
  wires:
  Detect Decrease/1 -> Falling_edge/1
  INPUT/1 -> Detect Decrease/1

== system tqd/TQD/TorqueDemand/Signal_convert/SWC_Subsystem/Speed Setting Mode/VTQD_SWCResUpPress_enum ==
  note: Long press or Short press
  INPUT : Inport
  task_time_s : Inport  Port=2
  AND : Logic  AllPortsSameDT=off  OutDataTypeStr=boolean
  AND1 : Logic  AllPortsSameDT=off  OutDataTypeStr=boolean
  Constant2 : Constant  Value=KTQD_SetSpdShortPLim_s
  Constant3 : Constant  Value=KTQD_SetSpdLongPLim_s
  Constant4 : Constant  Value=ENUM_SWCBOTTONPRESS_LONGPRESS
  Constant5 : Constant  Value=ENUM_SWCBOTTONPRESS_SHORTPRESS
  Constant6 : Constant  Value=ENUM_SWCBOTTONPRESS_NOPRESS
  Delay : Delay  DelayLength=1
  DelayEnable_LONG_PRESS1 : hcu_lib/Basic_Blocks/DelayEnable
  DelayEnable_SHORT_PRESS1 : hcu_lib/Basic_Blocks/DelayEnable
  Detect Decrease : simulink/Logic and Bit Operations/Detect Decrease  vinit=0.0  OutDataTypeStr=boolean
  Detect Decrease4 : simulink/Logic and Bit Operations/Detect Decrease  vinit=0.0  OutDataTypeStr=boolean
  NOT : Logic  Operator=NOT  AllPortsSameDT=off  OutDataTypeStr=boolean
  NOT1 : Logic  Operator=NOT  AllPortsSameDT=off  OutDataTypeStr=boolean
  SR_Latch : hcu_lib/Basic_Blocks/SR_Latch
  Switch : Switch  Criteria=u2 ~= 0
  Switch3 : Switch  Criteria=u2 ~= 0
  OUTPUT : Outport
  wires:
  [Short_press_falling_Edge] -> Switch3/2
  Detect Decrease/1 -> SR_Latch/2
  [INPUT] -> Detect Decrease/1
  NOT1/1 -> AND1/2
  SR_Latch/1 -> NOT1/1
  [INPUT] -> AND1/1
  AND1/1 -> DelayEnable_SHORT_PRESS1/1
  [Long_press_falling_edge] -> SR_Latch/1
  [INPUT] -> AND/1
  AND/1 -> DelayEnable_LONG_PRESS1/1
  NOT/1 -> AND/2
  Delay/1 -> NOT/1
  [Long_press_falling_edge] -> Delay/1
  INPUT/1 -> [INPUT]
  task_time_s/1 -> [task_time_s]
  DelayEnable_LONG_PRESS1/1 -> [Long_press_falling_edge]
  Switch3/1 -> Switch/3
  DelayEnable_SHORT_PRESS1/1 -> Detect Decrease4/1
  Constant3/1 -> DelayEnable_LONG_PRESS1/2
  Constant2/1 -> DelayEnable_SHORT_PRESS1/2
  [task_time_s] -> DelayEnable_SHORT_PRESS1/3
  [task_time_s] -> DelayEnable_LONG_PRESS1/3
  Detect Decrease4/1 -> [Short_press_falling_Edge]
  [Long_press_falling_edge] -> Switch/2
  Constant5/1 -> Switch3/1
  Constant4/1 -> Switch/1
  Constant6/1 -> Switch3/3
  Switch/1 -> OUTPUT/1

== system tqd/TQD/TorqueDemand/Signal_convert/SWC_Subsystem/Speed Setting Mode/VTQD_SWCSetDownPress_enum ==
  note: Long press or Short press
  INPUT : Inport
  task_time_s : Inport  Port=2
  AND : Logic  AllPortsSameDT=off  OutDataTypeStr=boolean
  AND1 : Logic  AllPortsSameDT=off  OutDataTypeStr=boolean
  Constant1 : Constant  Value=ENUM_SWCBOTTONPRESS_LONGPRESS
  Constant2 : Constant  Value=KTQD_SetSpdShortPLim_s
  Constant3 : Constant  Value=KTQD_SetSpdLongPLim_s
  Constant7 : Constant  Value=ENUM_SWCBOTTONPRESS_SHORTPRESS
  Constant8 : Constant  Value=ENUM_SWCBOTTONPRESS_NOPRESS
  Delay : Delay  DelayLength=1
  DelayEnable_LONG_PRESS1 : hcu_lib/Basic_Blocks/DelayEnable
  DelayEnable_SHORT_PRESS1 : hcu_lib/Basic_Blocks/DelayEnable
  Detect Decrease : simulink/Logic and Bit Operations/Detect Decrease  vinit=0.0  OutDataTypeStr=boolean
  Detect Decrease4 : simulink/Logic and Bit Operations/Detect Decrease  vinit=0.0  OutDataTypeStr=boolean
  NOT : Logic  Operator=NOT  AllPortsSameDT=off  OutDataTypeStr=boolean
  NOT1 : Logic  Operator=NOT  AllPortsSameDT=off  OutDataTypeStr=boolean
  SR_Latch : hcu_lib/Basic_Blocks/SR_Latch
  Switch : Switch  Criteria=u2 ~= 0
  Switch3 : Switch  Criteria=u2 ~= 0
  OUTPUT : Outport
  wires:
  [Short_press_falling_Edge] -> Switch3/2
  Detect Decrease/1 -> SR_Latch/2
  [INPUT] -> Detect Decrease/1
  NOT1/1 -> AND1/2
  SR_Latch/1 -> NOT1/1
  [INPUT] -> AND1/1
  AND1/1 -> DelayEnable_SHORT_PRESS1/1
  [Long_press_falling_edge] -> SR_Latch/1
  [INPUT] -> AND/1
  AND/1 -> DelayEnable_LONG_PRESS1/1
  NOT/1 -> AND/2
  Delay/1 -> NOT/1
  [Long_press_falling_edge] -> Delay/1
  INPUT/1 -> [INPUT]
  task_time_s/1 -> [task_time_s]
  DelayEnable_LONG_PRESS1/1 -> [Long_press_falling_edge]
  Switch3/1 -> Switch/3
  DelayEnable_SHORT_PRESS1/1 -> Detect Decrease4/1
  Constant3/1 -> DelayEnable_LONG_PRESS1/2
  Constant2/1 -> DelayEnable_SHORT_PRESS1/2
  [task_time_s] -> DelayEnable_SHORT_PRESS1/3
  [task_time_s] -> DelayEnable_LONG_PRESS1/3
  Detect Decrease4/1 -> [Short_press_falling_Edge]
  [Long_press_falling_edge] -> Switch/2
  Constant7/1 -> Switch3/1
  Constant1/1 -> Switch/1
  Constant8/1 -> Switch3/3
  Switch/1 -> OUTPUT/1

== system tqd/TQD/TorqueDemand/Signal_convert/VehWeightEst/Calaulation/Front Wheel Torque ==
  VINP_FrEDURealTMTq_Nm : Inport
  VTQD_VehWeightEstEn_flg : Inport  Port=2
  VTQD_VehWeightEstDis_flg : Inport  Port=3
  VTQD_VehWeightEstEnd_flg : Inport  Port=4
  task_time_s : Inport  Port=5
  AND : Logic  AllPortsSameDT=off  OutDataTypeStr=boolean
  AND1 : Logic  AllPortsSameDT=off  OutDataTypeStr=boolean
  AND2 : Logic  AllPortsSameDT=off  OutDataTypeStr=boolean
  Abs : Abs
  Add : Sum
  Add1 : Sum
  Add2 : Sum  Inputs=+-
  Constant1 : Constant  Value=ZERO_FLOAT
  Constant2 : Constant  Value=KTQD_VehWeighEstTime_s
  Constant3 : Constant  Value=ZERO_FLOAT
  Constant4 : Constant  Value=KTQD_VehWeighEstTimeTune_cnt
  Constant5 : Constant  Value=ZERO_FLOAT
  Constant6 : Constant  Value=KTQD_EstFrWhlTqDev_Nm
  Data Type Conversion : DataTypeConversion  OutDataTypeStr=uint8
  Delay{,1..4} (5 alike) : Delay  DelayLength=1
  Detect Decrease : simulink/Logic and Bit Operations/Detect Decrease  vinit=0.0  OutDataTypeStr=boolean
  Detect Increase : simulink/Logic and Bit Operations/Detect Increase  vinit=0.0  OutDataTypeStr=boolean
  Divide : Product  Inputs=*/
  Divide1 : Product  Inputs=*/
  Min : MinMax  Inputs=2
  NOT : Logic  Operator=NOT  AllPortsSameDT=off  OutDataTypeStr=boolean
  NOT1 : Logic  Operator=NOT  AllPortsSameDT=off  OutDataTypeStr=boolean
  Relational Operator : RelationalOperator  Operator=<=  OutDataTypeStr=boolean  RndMeth=Simplest
  Switch{,1..3} (4 alike) : Switch  Criteria=u2 > Threshold
  Terminator : Terminator
  VTQD_EstFrRealTqAvg_Nm : Outport
  VTQD_EstFrRealTqCheckPass_flg : Outport  Port=2
  wires:
  task_time_s/1 -> [task_time_s]
  VTQD_VehWeightEstEnd_flg/1 -> Terminator/1
  VTQD_VehWeightEstDis_flg/1 -> [VTQD_VehWeightEstDis_flg]
  VTQD_VehWeightEstEn_flg/1 -> [VTQD_VehWeightEstEn_flg]
  VINP_FrEDURealTMTq_Nm/1 -> [VINP_FrEDURealTMTq_Nm]
  AND1/1 -> [VTQD_EstFrRealTqCheckPass_flg]  "VTQD_EstFrRealTqCheckPass_flg"
  [VTQD_VehWeightEstDis_flg] -> AND1/1
  Add2/1 -> Abs/1
  Abs/1 -> Relational Operator/1
  Delay/1 -> NOT/1
  Detect Increase/1 -> Switch2/2
  [task_time_s] -> Divide/2
  [VTQD_EstFrRealTqMin_Nm] -> Delay2/1
  Delay2/1 -> Min/2
  [VTQD_VehWeightEstDis_flg] -> Delay/1
  [VTQD_EstFrRealTqMin_Nm] -> Add2/2
  Constant2/1 -> Divide/1
  Switch2/1 -> Delay4/1, [VTQD_EstFrRealTqMin_Nm]  "VTQD_EstFrRealTqMin_Nm"
  Add1/1 -> Divide1/2  "VTQD_EstCycleCount_cnt"
  Switch1/1 -> Delay1/1, [VTQD_EstFrRealTqSum_Nm]  "VTQD_EstFrRealTqSum_Nm"
  Constant5/1 -> Switch1/1
  NOT/1 -> AND/2
  [VINP_FrEDURealTMTq_Nm] -> Switch/1
  [VTQD_EstFrRealTqAvg_Nm] -> Add2/1
  Constant6/1 -> Relational Operator/2
  Add/1 -> Switch1/3
  Relational Operator/1 -> AND1/2
  [VTQD_VehWeightEstEn_flg] -> Detect Increase/1
  Constant1/1 -> Switch/3
  AND/1 -> Switch/2
  [VTQD_VehWeightEstEn_flg] -> Detect Decrease/1
  [VTQD_EstFrRealTqSum_Nm] -> Divide1/1
  Divide/1 -> Data Type Conversion/1
  Switch/1 -> Add/1
  Divide1/1 -> [VTQD_EstFrRealTqAvg_Nm]  "VTQD_EstFrRealTqAvg_Nm"
  [VTQD_VehWeightEstEn_flg] -> AND/1
  Constant3/1 -> Switch2/1
  Delay1/1 -> Add/2
  [VINP_FrEDURealTMTq_Nm] -> Min/1
  Constant4/1 -> Add1/2
  [VTQD_EstFrRealTqCheckPass_flg] -> VTQD_EstFrRealTqCheckPass_flg/1
  [VTQD_EstFrRealTqAvg_Nm] -> VTQD_EstFrRealTqAvg_Nm/1
  Data Type Conversion/1 -> Add1/1
  Delay3/1 -> NOT1/1
  [VTQD_VehWeightEstEn_flg] -> AND2/1
  AND2/1 -> Switch3/2
  NOT1/1 -> AND2/2
  [VTQD_VehWeightEstDis_flg] -> Delay3/1
  Delay4/1 -> Switch3/3
  Min/1 -> Switch3/1
  Switch3/1 -> Switch2/3
  Detect Decrease/1 -> Switch1/2

== system tqd/TQD/TorqueDemand/Signal_convert/VehWeightEst/Calaulation/Long Acc ==
  VVMC_LongAcc_Gps : Inport
  VTQD_VehWeightEstEn_flg : Inport  Port=2
  VTQD_VehWeightEstDis_flg : Inport  Port=3
  VTQD_VehWeightEstEnd_flg : Inport  Port=4
  task_time_s : Inport  Port=5
  AND : Logic  AllPortsSameDT=off  OutDataTypeStr=boolean
  AND1 : Logic  AllPortsSameDT=off  OutDataTypeStr=boolean
  AND2 : Logic  AllPortsSameDT=off  OutDataTypeStr=boolean
  Abs : Abs
  Abs1 : Abs
  Add : Sum
  Add1 : Sum
  Add2 : Sum  Inputs=+-
  Constant1 : Constant  Value=ZERO_FLOAT
  Constant2 : Constant  Value=KTQD_VehWeighEstTime_s
  Constant3 : Constant  Value=ZERO_FLOAT
  Constant4 : Constant  Value=KTQD_VehWeighEstTimeTune_cnt
  Constant5 : Constant  Value=ZERO_FLOAT
  Constant6 : Constant  Value=KTQD_EstLongAccDev_Gps
  Constant7 : Constant  Value=KTQD_VehWeighEstIntAcc_Gps
  Constant8 : Constant  Value=KTQD_VehWeighEstIntAcc_Gps
  Data Type Conversion : DataTypeConversion  OutDataTypeStr=uint8
  Delay{,1..4} (5 alike) : Delay  DelayLength=1
  Detect Decrease : simulink/Logic and Bit Operations/Detect Decrease  vinit=0.0  OutDataTypeStr=boolean
  Detect Increase : simulink/Logic and Bit Operations/Detect Increase  vinit=0.0  OutDataTypeStr=boolean
  Divide : Product  Inputs=*/
  Divide1 : Product  Inputs=*/
  Min : MinMax  Inputs=2
  NOT : Logic  Operator=NOT  AllPortsSameDT=off  OutDataTypeStr=boolean
  NOT1 : Logic  Operator=NOT  AllPortsSameDT=off  OutDataTypeStr=boolean
  Relational Operator : RelationalOperator  Operator=<=  OutDataTypeStr=boolean  RndMeth=Simplest
  Relational Operator1 : RelationalOperator  Operator=<=  OutDataTypeStr=boolean  RndMeth=Simplest
  Switch{,1..4} (5 alike) : Switch  Criteria=u2 > Threshold
  Terminator : Terminator
  VTQD_EstLongAccAvg_Gps : Outport
  VTQD_EstLongAccCheckPass_flg : Outport  Port=2
  wires:
  Constant4/1 -> Add1/2
  [VVMC_LongAcc_Gps] -> Min/1
  Delay1/1 -> Add/2
  Constant3/1 -> Switch2/1
  [VTQD_VehWeightEstEn_flg] -> AND/1
  Divide1/1 -> [VTQD_EstLongAccAvg_Gps]  "VTQD_EstLongAccAvg_Gps"
  Switch/1 -> Add/1
  Data Type Conversion/1 -> Add1/1
  AND/1 -> Switch/2
  Constant1/1 -> Switch/3
  [VTQD_VehWeightEstEn_flg] -> Detect Increase/1
  Relational Operator/1 -> AND1/2
  Divide/1 -> Data Type Conversion/1
  Add/1 -> Switch1/3
  Constant6/1 -> Relational Operator/2
  [VTQD_EstLongAccAvg_Gps] -> Add2/1
  [VVMC_LongAcc_Gps] -> Switch/1
  NOT/1 -> AND/2
  Constant5/1 -> Switch1/1
  Switch1/1 -> [VTQD_EstLongAccSum_Gps], Delay1/1  "VTQD_EstLongAccSum_Gps"
  Add1/1 -> Divide1/2  "VTQD_EstCycleCount_cnt"
  Switch2/1 -> Delay4/1, [VTQD_EstLongAccMin_Gps]  "VTQD_EstLongAccMin_Gps"
  Constant2/1 -> Divide/1
  [VTQD_EstLongAccMin_Gps] -> Add2/2
  [VTQD_VehWeightEstDis_flg] -> Delay/1
  Delay2/1 -> Min/2
  [VTQD_EstLongAccMin_Gps] -> Delay2/1
  [task_time_s] -> Divide/2
  Detect Increase/1 -> Switch2/2
  Delay/1 -> NOT/1
  Abs/1 -> Relational Operator/1
  Add2/1 -> Abs/1
  [VTQD_VehWeightEstDis_flg] -> AND1/1
  AND1/1 -> [VTQD_EstLongAccCheckPass_flg]  "VTQD_EstLongAccCheckPass_flg"
  VVMC_LongAcc_Gps/1 -> [VVMC_LongAcc_Gps]
  VTQD_VehWeightEstEn_flg/1 -> [VTQD_VehWeightEstEn_flg]
  VTQD_VehWeightEstDis_flg/1 -> [VTQD_VehWeightEstDis_flg]
  VTQD_VehWeightEstEnd_flg/1 -> Terminator/1
  task_time_s/1 -> [task_time_s]
  [VTQD_EstLongAccAvg_Gps] -> VTQD_EstLongAccAvg_Gps/1
  [VTQD_EstLongAccCheckPass_flg] -> VTQD_EstLongAccCheckPass_flg/1
  AND2/1 -> Switch3/2
  [VTQD_VehWeightEstDis_flg] -> Delay3/1
  NOT1/1 -> AND2/2
  [VTQD_VehWeightEstEn_flg] -> AND2/1
  Delay3/1 -> NOT1/1
  Min/1 -> Switch3/1
  Delay4/1 -> Switch3/3
  Switch3/1 -> Switch2/3
  Detect Decrease/1 -> Switch1/2
  [VTQD_VehWeightEstEn_flg] -> Detect Decrease/1
  [VTQD_EstLongAccSum_Gps] -> Switch4/3
  Switch4/1 -> Divide1/1
  [VTQD_EstLongAccSum_Gps] -> Abs1/1
  Abs1/1 -> Relational Operator1/1
  Relational Operator1/1 -> Switch4/2
  Constant7/1 -> Relational Operator1/2
  Constant8/1 -> Switch4/1

== system tqd/TQD/TorqueDemand/Signal_convert/VehWeightEst/Calaulation/Rear Wheel Torque ==
  VINP_RrEDURealTMTq_Nm : Inport
  VTQD_VehWeightEstEn_flg : Inport  Port=2
  VTQD_VehWeightEstDis_flg : Inport  Port=3
  VTQD_VehWeightEstEnd_flg : Inport  Port=4
  task_time_s : Inport  Port=5
  AND : Logic  AllPortsSameDT=off  OutDataTypeStr=boolean
  AND1 : Logic  AllPortsSameDT=off  OutDataTypeStr=boolean
  AND2 : Logic  AllPortsSameDT=off  OutDataTypeStr=boolean
  Abs : Abs
  Add : Sum
  Add1 : Sum
  Add2 : Sum  Inputs=+-
  Constant1 : Constant  Value=ZERO_FLOAT
  Constant2 : Constant  Value=KTQD_VehWeighEstTime_s
  Constant3 : Constant  Value=ZERO_FLOAT
  Constant4 : Constant  Value=KTQD_VehWeighEstTimeTune_cnt
  Constant5 : Constant  Value=ZERO_FLOAT
  Constant6 : Constant  Value=KTQD_EstRrWhlTqDev_Nm
  Data Type Conversion : DataTypeConversion  OutDataTypeStr=uint8
  Delay{,1..4} (5 alike) : Delay  DelayLength=1
  Detect Decrease : simulink/Logic and Bit Operations/Detect Decrease  vinit=0.0  OutDataTypeStr=boolean
  Detect Increase : simulink/Logic and Bit Operations/Detect Increase  vinit=0.0  OutDataTypeStr=boolean
  Divide : Product  Inputs=*/
  Divide1 : Product  Inputs=*/
  Min : MinMax  Inputs=2
  NOT : Logic  Operator=NOT  AllPortsSameDT=off  OutDataTypeStr=boolean
  NOT1 : Logic  Operator=NOT  AllPortsSameDT=off  OutDataTypeStr=boolean
  Relational Operator : RelationalOperator  Operator=<=  OutDataTypeStr=boolean  RndMeth=Simplest
  Switch{,1..3} (4 alike) : Switch  Criteria=u2 > Threshold
  Terminator : Terminator
  VTQD_EstRrRealTqAvg_Nm : Outport
  VTQD_EstRrRealTqCheckPass_flg : Outport  Port=2
  wires:
  [VTQD_EstRrRealTqAvg_Nm] -> VTQD_EstRrRealTqAvg_Nm/1
  [VTQD_EstRrRealTqCheckPass_flg] -> VTQD_EstRrRealTqCheckPass_flg/1
  Constant4/1 -> Add1/2
  [VINP_RrEDURealTMTq_Nm] -> Min/1
  Delay1/1 -> Add/2
  Constant3/1 -> Switch2/1
  [VTQD_VehWeightEstEn_flg] -> AND/1
  Divide1/1 -> [VTQD_EstRrRealTqAvg_Nm]  "VTQD_EstRrRealTqAvg_Nm"
  Switch/1 -> Add/1
  [VTQD_EstRrRealTqSum_Nm] -> Divide1/1
  [VTQD_VehWeightEstEn_flg] -> Detect Decrease/1
  AND/1 -> Switch/2
  Constant1/1 -> Switch/3
  [VTQD_VehWeightEstEn_flg] -> Detect Increase/1
  Relational Operator/1 -> AND1/2
  Add/1 -> Switch1/3
  Constant6/1 -> Relational Operator/2
  [VTQD_EstRrRealTqAvg_Nm] -> Add2/1
  [VINP_RrEDURealTMTq_Nm] -> Switch/1
  NOT/1 -> AND/2
  Constant5/1 -> Switch1/1
  Switch1/1 -> [VTQD_EstRrRealTqSum_Nm], Delay1/1  "VTQD_EstRrRealTqSum_Nm"
  Switch2/1 -> Delay4/1, [VTQD_EstRrRealTqMin_Nm]  "VTQD_EstRrRealTqMin_Nm"
  Constant2/1 -> Divide/1
  [VTQD_EstRrRealTqMin_Nm] -> Add2/2
  [VTQD_VehWeightEstDis_flg] -> Delay/1
  Delay2/1 -> Min/2
  [VTQD_EstRrRealTqMin_Nm] -> Delay2/1
  [task_time_s] -> Divide/2
  Detect Increase/1 -> Switch2/2
  Delay/1 -> NOT/1
  Abs/1 -> Relational Operator/1
  Add2/1 -> Abs/1
  [VTQD_VehWeightEstDis_flg] -> AND1/1
  AND1/1 -> [VTQD_EstRrRealTqCheckPass_flg]  "VTQD_EstRrRealTqCheckPass_flg"
  VINP_RrEDURealTMTq_Nm/1 -> [VINP_RrEDURealTMTq_Nm]
  VTQD_VehWeightEstEn_flg/1 -> [VTQD_VehWeightEstEn_flg]
  VTQD_VehWeightEstDis_flg/1 -> [VTQD_VehWeightEstDis_flg]
  VTQD_VehWeightEstEnd_flg/1 -> Terminator/1
  task_time_s/1 -> [task_time_s]
  Add1/1 -> Divide1/2  "VTQD_EstCycleCount_cnt"
  Divide/1 -> Data Type Conversion/1
  Data Type Conversion/1 -> Add1/1
  [VTQD_VehWeightEstEn_flg] -> AND2/1
  NOT1/1 -> AND2/2
  Delay3/1 -> NOT1/1
  [VTQD_VehWeightEstDis_flg] -> Delay3/1
  AND2/1 -> Switch3/2
  Min/1 -> Switch3/1
  Switch3/1 -> Switch2/3
  Delay4/1 -> Switch3/3
  Detect Decrease/1 -> Switch1/2

== system tqd/TQD/TorqueDemand/Signal_convert/VehWeightEst/Calaulation/Vehicle Weight ==
  VTQD_EstFrRealTqAvg_Nm : Inport
  VTQD_EstRrRealTqAvg_Nm : Inport  Port=2
  VTQD_EstLongAccAvg_Gps : Inport  Port=3
  VINP_VehSpeed_kph : Inport  Port=4
  Add : Sum  Inputs=+++
  Add1 : Sum
  Add2 : Sum
  Add3 : Sum
  Constant1 : Constant  Value=KTQD_RrTMTotalGearRatio_gain
  Constant10 : Constant  Value=KTQR_FrTMGearEff_c
  Constant11 : Constant  Value=KTQR_RrTMGearEff_c
  Constant12 : Constant  Value=MINUSONE_FLOAT
  Constant13 : Constant  Value=KTQD_GravityValue_mps2
  Constant2 : Constant  Value=KTQD_FrTMTotalGearRatio_gain
  Constant3 : Constant  Value=MINUSONE_FLOAT
  Constant4 : Constant  Value=MINUSONE_FLOAT
  Constant5 : Constant  Value=KTQD_FrTireRadius_m
  Constant6 : Constant  Value=KTQD_RrTireRadius_m
  Constant7 : Constant  Value=KTQD_EstRollCoeffA_c
  Constant8 : Constant  Value=KTQD_EstRollCoeffB_c
  Constant9 : Constant  Value=KTQD_EstRollCoeffC_c
  Divide : Product  Inputs=*/
  Divide1 : Product  Inputs=*/
  Divide2 : Product  Inputs=*/
  Product{,3..5} (4 alike) : Product
  Product1 : Product  Inputs=3
  Product2 : Product  Inputs=3
  Product6 : Product  Inputs=3
  Square : Math  Operator=square  SaturateOnIntegerOverflow=on
  VTQD_EstVehWeight_kg : Outport
  wires:
  [VINP_VehSpeed_kph] -> Square/1
  Divide/1 -> Add1/1  "VTQD_EstFrForce_N"
  Product2/1 -> Divide2/1  "VTQD_EstRrWhlTqAvg_Nm"
  [VINP_VehSpeed_kph] -> Product/2
  Constant6/1 -> Divide2/2
  Product1/1 -> Divide/1  "VTQD_EstFrWhlTqAvg_Nm"
  Constant2/1 -> Product1/2
  Constant1/1 -> Product2/2
  Add1/1 -> Product4/1
  Square/1 -> Product3/2
  [VTQD_EstRrRealTqAvg_Nm] -> Product2/1
  Constant3/1 -> Product1/3
  [VTQD_EstRollForce_N] -> Add2/2
  Constant9/1 -> Product3/1
  Constant7/1 -> Add/1
  [VTQD_EstFrRealTqAvg_Nm] -> Product1/1
  Constant10/1 -> Product4/2
  Add2/1 -> Product5/1
  Product4/1 -> Add3/1  "VTQD_EstFrActForce_N"
  Constant5/1 -> Divide/2
  Add/1 -> [VTQD_EstRollForce_N]  "VTQD_EstRollForce_N"
  Product/1 -> Add/2
  Constant4/1 -> Product2/3
  Add3/1 -> [VTQD_EstActTotalForce_N]  "VTQD_EstActTotalForce_N"
  Product5/1 -> Add3/2  "VTQD_EstRrActForce_N"
  Constant8/1 -> Product/1
  Divide2/1 -> Add2/1  "VTQD_EstRrForce_N"
  Constant11/1 -> Product5/2
  [VTQD_EstRollForce_N] -> Add1/2
  Product3/1 -> Add/3
  [VTQD_EstLongAccAvg_Gps] -> Product6/1
  Constant12/1 -> Product6/2
  Product6/1 -> Divide1/2
  [VTQD_EstActTotalForce_N] -> Divide1/1
  VTQD_EstFrRealTqAvg_Nm/1 -> [VTQD_EstFrRealTqAvg_Nm]
  VTQD_EstRrRealTqAvg_Nm/1 -> [VTQD_EstRrRealTqAvg_Nm]
  VTQD_EstLongAccAvg_Gps/1 -> [VTQD_EstLongAccAvg_Gps]
  VINP_VehSpeed_kph/1 -> [VINP_VehSpeed_kph]
  [VTQD_EstVehWeight_kg] -> VTQD_EstVehWeight_kg/1
  Constant13/1 -> Product6/3
  Divide1/1 -> [VTQD_EstVehWeight_kg]  "VTQD_EstVehWeight_kg"
